simulink model "Virtual_Engine_Combustion_Model"  (R2016b)
settings: Solver=FixedStepDiscrete  StartTime=0.0  StopTime=inf  FixedStep=VirtEngCmbMdl.tiSimnTiStep_C  RelTol=1e-3  EnableMultiTasking=on
settings Model: Creator=m01wolf  LastModifiedBy=bunver
settings DataIOCC: SaveFormat=StructureWithTime  SaveOutput=off  DSMLogging=off  VisualizeSimOutput=off  SaveTime=off  StateSaveName=Results  SignalLoggingName=Results
settings OptimizationCC: BlockReduction=off  ConditionallyExecuteInputs=off  LifeSpan=inf
settings DebuggingCC: AllowSymbolicDim=off  SFUnexpectedBacktrackingDiag=warning  SFNoUnconditionalDefaultTransitionDiag=warning  SFExecutionAtInitializationDiag=none
settings ModelReferenceCC: ModelReferenceNumInstancesAllowed=Single  PropagateSignalLabelsOutOfModel=off
settings GRTTargetCC: TargetLangStandard=C89/C90 (ANSI)
settings ConfigComp: CovMetricSettings=dw  CovHtmlReporting=on  CovSaveCumulativeToWorkspaceVar=on  CovSaveSingleToWorkspaceVar=on  CovExternalEMLEnable=off

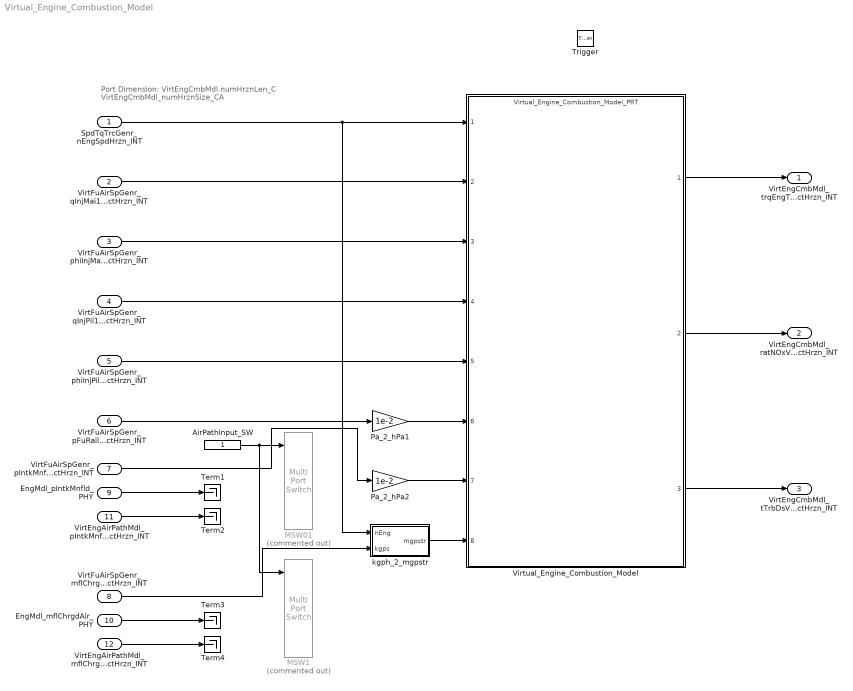
== system Virtual_Engine_Combustion_Model ==
  note: Port Dimension: VirtEngCmbMdl.numHrznLen_C
      | VirtEngCmbMdl_numHrznSize_CA
  SpdTqTrcGenr_nEngSpdHrzn_INT : Inport  PortDimensions=VirtEngCmbMdl_numHrznSize_CA
  VirtFuAirSpGenr_qInjMai1VectHrzn_INT : Inport  Port=2  PortDimensions=VirtEngCmbMdl_numHrznSize_CA
  VirtFuAirSpGenr_phiInjMai1VectHrzn_INT : Inport  Port=3  PortDimensions=VirtEngCmbMdl_numHrznSize_CA
  VirtFuAirSpGenr_qInjPil1VectHrzn_INT : Inport  Port=4  PortDimensions=VirtEngCmbMdl_numHrznSize_CA
  VirtFuAirSpGenr_phiInjPil1VectHrzn_INT : Inport  Port=5  PortDimensions=VirtEngCmbMdl_numHrznSize_CA
  VirtFuAirSpGenr_pFuRailDesVectHrzn_INT : Inport  Port=6  PortDimensions=VirtEngCmbMdl_numHrznSize_CA
  VirtFuAirSpGenr_pIntkMnfldDesVectHrzn_INT : Inport  Port=7  PortDimensions=VirtEngCmbMdl_numHrznSize_CA
  VirtFuAirSpGenr_mflChrgdAirDesVectHrzn_INT : Inport  Port=8  PortDimensions=VirtEngCmbMdl_numHrznSize_CA
  EngMdl_pIntkMnfld_PHY : Inport  Port=9
  EngMdl_mflChrgdAir_PHY : Inport  Port=10
  VirtEngAirPathMdl_pIntkMnfldVectHrzn_INT : Inport  Port=11  PortDimensions=VirtEngCmbMdl_numHrznSize_CA
  VirtEngAirPathMdl_mflChrgdAirVectHrzn_INT : Inport  Port=12  PortDimensions=VirtEngCmbMdl_numHrznSize_CA
  Trigger : TriggerPort  TriggerType=function-call  VariantControl=Variant  PortDimensions=1
  AirPathInput_SW : Constant  SampleTime=-1
  MSW01 : MultiPortSwitch  Commented=on
  MSW1 : MultiPortSwitch  Commented=on
  Pa_2_hPa1 : Gain  Gain=1e-2
  Pa_2_hPa2 : Gain  Gain=1e-2
  Term{1..4} (4 alike) : Terminator
  Virtual_Engine_Combustion_Model : ModelReference  ModelNameDialog=Virtual_Engine_Combustion_Model_PRT.slxp  ModelReferenceVersion=1.276  CopyOfModelProtected=on
  kgph_2_mgpstr : Subsystem
  VirtEngCmbMdl_trqEngTqOutVectHrzn_INT : Outport
  VirtEngCmbMdl_ratNOxVectHrzn_INT : Outport  Port=2
  VirtEngCmbMdl_tTrbDsVectHrzn_INT : Outport  Port=3
  wires:
  Pa_2_hPa1/1 -> Virtual_Engine_Combustion_Model/6
  Pa_2_hPa2/1 -> Virtual_Engine_Combustion_Model/7
  VirtFuAirSpGenr_pIntkMnfldDesVectHrzn_INT/1 -> Pa_2_hPa2/1
  VirtFuAirSpGenr_mflChrgdAirDesVectHrzn_INT/1 -> kgph_2_mgpstr/2(kgps)
  AirPathInput_SW/1 -> MSW1/1, MSW01/1
  kgph_2_mgpstr/1(mgpstr) -> Virtual_Engine_Combustion_Model/8
  VirtEngAirPathMdl_pIntkMnfldVectHrzn_INT/1 -> Term2/1
  SpdTqTrcGenr_nEngSpdHrzn_INT/1 -> Virtual_Engine_Combustion_Model/1, kgph_2_mgpstr/1(nEng)
  VirtFuAirSpGenr_qInjMai1VectHrzn_INT/1 -> Virtual_Engine_Combustion_Model/2
  VirtFuAirSpGenr_phiInjMai1VectHrzn_INT/1 -> Virtual_Engine_Combustion_Model/3
  VirtFuAirSpGenr_qInjPil1VectHrzn_INT/1 -> Virtual_Engine_Combustion_Model/4
  VirtFuAirSpGenr_phiInjPil1VectHrzn_INT/1 -> Virtual_Engine_Combustion_Model/5
  VirtFuAirSpGenr_pFuRailDesVectHrzn_INT/1 -> Pa_2_hPa1/1
  EngMdl_mflChrgdAir_PHY/1 -> Term3/1
  EngMdl_pIntkMnfld_PHY/1 -> Term1/1
  VirtEngAirPathMdl_mflChrgdAirVectHrzn_INT/1 -> Term4/1
  Virtual_Engine_Combustion_Model/1 -> VirtEngCmbMdl_trqEngTqOutVectHrzn_INT/1
  Virtual_Engine_Combustion_Model/2 -> VirtEngCmbMdl_ratNOxVectHrzn_INT/1
  Virtual_Engine_Combustion_Model/3 -> VirtEngCmbMdl_tTrbDsVectHrzn_INT/1

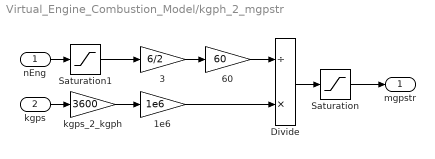
== system Virtual_Engine_Combustion_Model/kgph_2_mgpstr ==
  nEng : Inport
  kgps : Inport  Port=2
  1e6 : Gain  Gain=1e6
  3 : Gain  Gain=6/2
  60 : Gain  Gain=60
  Divide : Product  Inputs=/*
  Saturation : Saturate  UpperLimit=inf  LowerLimit=0
  Saturation1 : Saturate  UpperLimit=inf  LowerLimit=300
  kgps_2_kgph : Gain  Gain=3600
  mgpstr : Outport
  wires:
  Saturation1/1 -> 3/1
  Divide/1 -> Saturation/1
  nEng/1 -> Saturation1/1
  kgps/1 -> kgps_2_kgph/1
  Saturation/1 -> mgpstr/1
  kgps_2_kgph/1 -> 1e6/1
  1e6/1 -> Divide/2
  3/1 -> 60/1
  60/1 -> Divide/1
